simulink model "Assemble_Blocks_Aug_10"  (R2019a)
settings: Solver=VariableStepAuto  StartTime=0.0  StopTime=10.0  RelTol=1e-3
libraries: sailbot_library x19
settings Model: Creator=tylerlum  LastModifiedBy=tylerlum

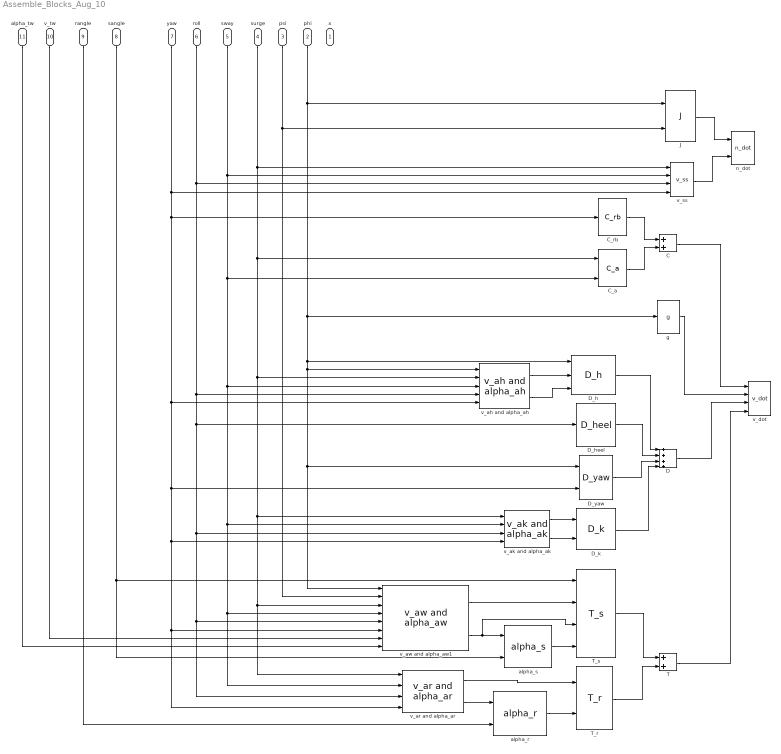
== system Assemble_Blocks_Aug_10 ==
  x : Inport
  phi : Inport  Port=2
  psi : Inport  Port=3
  surge : Inport  Port=4
  sway : Inport  Port=5
  roll : Inport  Port=6
  yaw : Inport  Port=7
  sangle : Inport  Port=8
  rangle : Inport  Port=9
  v_tw : Inport  Port=10
  alpha_tw : Inport  Port=11
  C : Sum
  C_a : sailbot_library/C_a  SystemSampleTime=-1
  C_rb : sailbot_library/C_rb  SystemSampleTime=-1
  D : Sum  Inputs=4
  D_h : sailbot_library/D_h  SystemSampleTime=-1
  "D_heel " : sailbot_library/D_heel   SystemSampleTime=-1
  D_k : sailbot_library/D_k  SystemSampleTime=-1
  D_yaw : sailbot_library/D_yaw  SystemSampleTime=-1
  J : sailbot_library/J  SystemSampleTime=-1
  T : Sum
  T_r : sailbot_library/T_r  SystemSampleTime=-1
  "T_s " : sailbot_library/T_s   SystemSampleTime=-1
  alpha_r : sailbot_library/alpha_r  SystemSampleTime=-1
  alpha_s : sailbot_library/alpha_s  SystemSampleTime=-1
  g : sailbot_library/g  SystemSampleTime=-1
  n_dot : sailbot_library/n_dot  SystemSampleTime=-1
  v_ah and alpha_ah : sailbot_library/v_ah and alpha_ah  SystemSampleTime=-1
  v_ak and alpha_ak : sailbot_library/v_ak and alpha_ak  SystemSampleTime=-1
  v_ar and alpha_ar : sailbot_library/v_ar and alpha_ar  SystemSampleTime=-1
  v_aw and alpha_aw1 : sailbot_library/v_aw and alpha_aw  SystemSampleTime=-1
  v_dot : sailbot_library/v_dot  SystemSampleTime=-1
  v_ss : sailbot_library/v_ss  SystemSampleTime=-1
  wires:
  C_rb/1 -> C/1
  C_a/1 -> C/2
  J/1 -> n_dot/1
  v_ss/1 -> n_dot/2
  C/1 -> v_dot/1
  "T_s "/1 -> T/1
  T_r/1 -> T/2
  T/1 -> v_dot/4
  alpha_s/1 -> "T_s "/4
  alpha_r/1 -> T_r/2
  v_ar and alpha_ar/2 -> alpha_r/1
  v_ar and alpha_ar/1 -> T_r/1
  v_aw and alpha_aw1/1 -> "T_s "/2
  v_aw and alpha_aw1/2 -> "T_s "/3, alpha_s/1
  D_h/1 -> D/1
  "D_heel "/1 -> D/2
  D_yaw/1 -> D/3
  D/1 -> v_dot/3
  g/1 -> v_dot/2
  v_ah and alpha_ah/1 -> D_h/2
  v_ah and alpha_ah/2 -> D_h/3
  D_k/1 -> D/4
  v_ak and alpha_ak/1 -> D_k/1
  v_ak and alpha_ak/2 -> D_k/2
  rangle/1 -> alpha_r/2
  yaw/1 -> v_ss/4, D_yaw/2, v_ak and alpha_ak/4, v_ar and alpha_ar/4, v_aw and alpha_aw1/6, v_ah and alpha_ah/5, C_rb/1
  roll/1 -> v_ss/3, v_ah and alpha_ah/4, "D_heel "/1, v_ak and alpha_ak/3, v_aw and alpha_aw1/5, v_ar and alpha_ar/3
  sway/1 -> v_ss/2, C_a/2, v_ah and alpha_ah/3, v_aw and alpha_aw1/4, v_ar and alpha_ar/2, v_ak and alpha_ak/2
  surge/1 -> v_ak and alpha_ak/1, v_aw and alpha_aw1/3, v_ar and alpha_ar/1, v_ah and alpha_ah/2, C_a/1, v_ss/1
  sangle/1 -> "T_s "/1, alpha_s/2
  alpha_tw/1 -> v_aw and alpha_aw1/8
  v_tw/1 -> v_aw and alpha_aw1/7
  psi/1 -> v_aw and alpha_aw1/2, J/2
  phi/1 -> J/1, D_h/1, D_yaw/1, v_aw and alpha_aw1/1, v_ah and alpha_ah/1, g/1
